simulink model "lab3Sim"  (Simulink 7.1)
settings: Solver=ode45  StartTime=0.0  StopTime=50  RelTol=1e-3
settings Model: Creator=CARLOS BRUNO  LastModifiedBy=CARLOS BRUNO

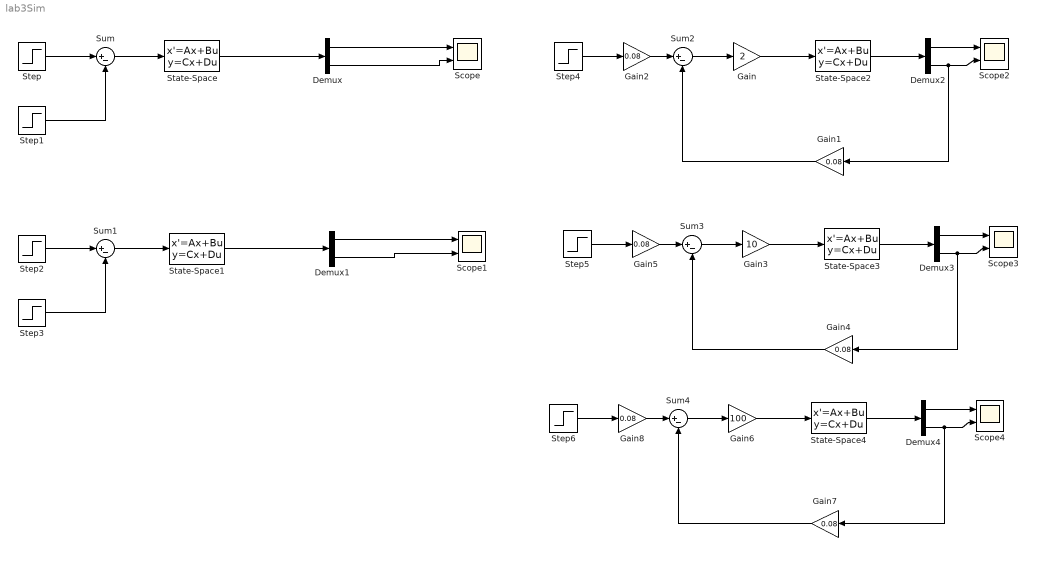
== system lab3Sim ==
  Demux{,1..4} (5 alike) : Demux  Outputs=2
  Gain : Gain  Gain=2  ParameterDataType=sfix(16)  ParameterScaling=2^0  OutDataType=sfix(16)  OutScaling=2^0
  Gain1 : Gain  Orientation=left  Gain=0.08  ParameterDataType=sfix(16)  ParameterScaling=2^0  OutDataType=sfix(16)  OutScaling=2^0
  Gain2 : Gain  Gain=0.08  ParameterDataType=sfix(16)  ParameterScaling=2^0  OutDataType=sfix(16)  OutScaling=2^0
  Gain3 : Gain  Gain=10  ParameterDataType=sfix(16)  ParameterScaling=2^0  OutDataType=sfix(16)  OutScaling=2^0
  Gain4 : Gain  Orientation=left  Gain=0.08  ParameterDataType=sfix(16)  ParameterScaling=2^0  OutDataType=sfix(16)  OutScaling=2^0
  Gain5 : Gain  Gain=0.08  ParameterDataType=sfix(16)  ParameterScaling=2^0  OutDataType=sfix(16)  OutScaling=2^0
  Gain6 : Gain  Gain=100  ParameterDataType=sfix(16)  ParameterScaling=2^0  OutDataType=sfix(16)  OutScaling=2^0
  Gain7 : Gain  Orientation=left  Gain=0.08  ParameterDataType=sfix(16)  ParameterScaling=2^0  OutDataType=sfix(16)  OutScaling=2^0
  Gain8 : Gain  Gain=0.08  ParameterDataType=sfix(16)  ParameterScaling=2^0  OutDataType=sfix(16)  OutScaling=2^0
  Scope{,1..4} (5 alike) : Scope  NumInputPorts=2
      Scope settings: YMin=-5~-5  YMax=5~5
      Scope1 settings: YMin=-5~-5  YMax=5~5
      Scope2 settings: YMin=-5~-5  YMax=5~5  SaveName=ScopeData2
      Scope3 settings: YMin=-5~-5  YMax=5~5  SaveName=ScopeData3
      Scope4 settings: YMin=-5~-5  YMax=5~5  SaveName=ScopeData4
  State-Space{,2..4} (4 alike) : StateSpace  A=[-250 -0.4 0; 1.1962 -0.0268 0; 0 1.0 0]  B=[5.0; 0; 0]  C=[0 0.1 0; 0 0 0.1 ]  D=[0;0]
  State-Space1 : StateSpace  A=[-250 -0.4 0; 1.2103 -0.0259 0; 0 1 0]  B=[5.0; 0; 0]  C=[0 1 0; 0 0 1 ]  D=[0;0]
  Step : Step  Time=0  After=12  SampleTime=0
  Step1 : Step  Time=10  After=12  SampleTime=0
  Step2 : Step  Time=0  After=12  SampleTime=0
  Step3 : Step  Time=10  After=12  SampleTime=0
  Step4 : Step  Time=0  After=pi/3  SampleTime=0
  Step5 : Step  Time=0  After=pi/3  SampleTime=0
  Step6 : Step  Time=0  After=pi/3  SampleTime=0
  Sum{,1..4} (5 alike) : Sum  Inputs=|+-  OutDataType=sfix(16)  OutScaling=2^0
  wires:
  Step/1 -> Sum/1
  Sum/1 -> State-Space/1
  State-Space/1 -> Demux/1
  Step1/1 -> Sum/2
  Step2/1 -> Sum1/1
  Step3/1 -> Sum1/2
  Sum1/1 -> State-Space1/1
  State-Space1/1 -> Demux1/1
  Demux1/2 -> Scope1/2
  Demux1/1 -> Scope1/1
  Demux/2 -> Scope/2
  Demux/1 -> Scope/1
  State-Space2/1 -> Demux2/1
  Demux2/2 -> Scope2/2, Gain1/1
  Demux2/1 -> Scope2/1
  Gain/1 -> State-Space2/1
  Step4/1 -> Gain2/1
  Gain2/1 -> Sum2/1
  Sum2/1 -> Gain/1
  Gain1/1 -> Sum2/2
  State-Space3/1 -> Demux3/1
  Demux3/2 -> Scope3/2, Gain4/1
  Demux3/1 -> Scope3/1
  Gain3/1 -> State-Space3/1
  Step5/1 -> Gain5/1
  Gain5/1 -> Sum3/1
  Sum3/1 -> Gain3/1
  Gain4/1 -> Sum3/2
  State-Space4/1 -> Demux4/1
  Demux4/2 -> Scope4/2, Gain7/1
  Demux4/1 -> Scope4/1
  Gain6/1 -> State-Space4/1
  Step6/1 -> Gain8/1
  Gain8/1 -> Sum4/1
  Sum4/1 -> Gain6/1
  Gain7/1 -> Sum4/2
